simulink model "Swerve_Drive_Example_Model"  (R2023a)
settings: Solver=daessc  StartTime=0.0  StopTime=20  FixedStep=t_sample  RelTol=1e-3
undefined symbols (not defined in the file): t_sample
libraries: Swerve_Modules_Controls_Lib x2, SignalEditorBlockLib x1, Simulation_lib x1
settings Model: SimulationMode=accelerator  Creator=ander  LastModifiedBy=ander

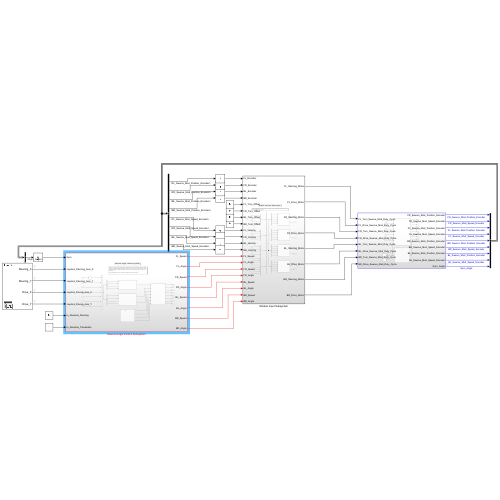
[thumbnail: Simulink's stored preview of the top-level diagram]
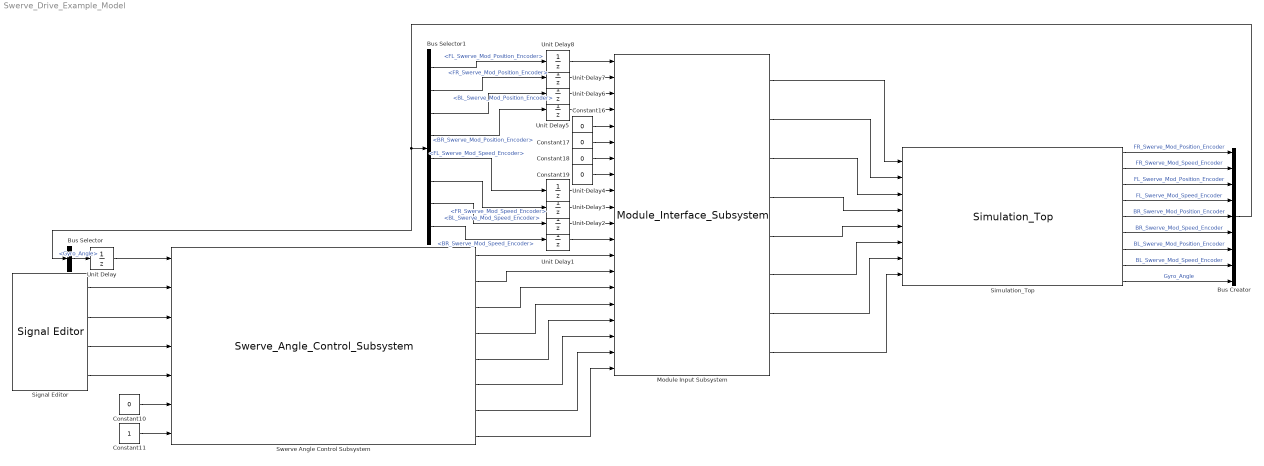
== system Swerve_Drive_Example_Model ==
  Bus Creator : BusCreator  Inputs=9
  Bus Selector : BusSelector  OutputSignals=Gyro_Angle
  Bus Selector1 : BusSelector  OutputSignals=FL_Swerve_Mod_Position_Encoder,FR_Swerve_Mod_Position_Encoder,BL_Swerve_Mod_Position_Encoder,BR_Swerve_Mod_Position_Encoder,FL_Swerve_Mod_Speed_Encoder,FR_Swerve_Mod_Speed_Encoder,BL_Swerve_Mod_Speed_Encoder,BR_Swerve_Mod_Speed_Encoder
  Constant10 : Constant  Value=0  OutDataTypeStr=boolean
  Constant11 : Constant  OutDataTypeStr=boolean
  Constant{16..19} (4 alike) : Constant  Value=0
  Module Input Subsystem : Swerve_Modules_Controls_Lib/Module_Interface_Subsystem  SystemSampleTime=-1  VariantActivationTime=update diagram  Latency=0  AutoFrameSizeCalculation=off
  Signal Editor : SignalEditorBlockLib/Signal Editor  FileName=C:\Users\ander\MATLAB\Projects\SwervePuppy-2.0-VSCODE\simulink\Unit_Tests\Joystick_input_test_data.mat  ActiveScenario=TempTest  ActiveSignal=Drive_X  IsBus=off  OutputBusObjectStr=Bus: BusObject  SampleTime=t_sample  ZeroCross=off  OutputAfterFinalValue=Setting to zero  Unit=inherit  PreserveSignalName=on  ApplySigPropsToAllScenarios=on
  Simulation_Top : Simulation_lib/Simulation_Top  SystemSampleTime=-1  VariantActivationTime=update diagram  Latency=0  AutoFrameSizeCalculation=off
  Swerve Angle Control Subsystem : Swerve_Modules_Controls_Lib/Swerve_Angle_Control_Subsystem  SystemSampleTime=-1  VariantActivationTime=update diagram  Latency=0  AutoFrameSizeCalculation=off
  Unit Delay{,1..8} (9 alike) : UnitDelay  SampleTime=-1  HasFrameUpgradeWarning=on
  wires:
  Constant11/1 -> Swerve Angle Control Subsystem/7
  Constant10/1 -> Swerve Angle Control Subsystem/6
  Constant17/1 -> Module Input Subsystem/6
  Constant19/1 -> Module Input Subsystem/8
  Constant16/1 -> Module Input Subsystem/5
  Constant18/1 -> Module Input Subsystem/7
  Swerve Angle Control Subsystem/4 -> Module Input Subsystem/16
  Swerve Angle Control Subsystem/6 -> Module Input Subsystem/18
  Swerve Angle Control Subsystem/7 -> Module Input Subsystem/19
  Swerve Angle Control Subsystem/2 -> Module Input Subsystem/14
  Swerve Angle Control Subsystem/8 -> Module Input Subsystem/20
  Swerve Angle Control Subsystem/3 -> Module Input Subsystem/15
  Swerve Angle Control Subsystem/1 -> Module Input Subsystem/13
  Swerve Angle Control Subsystem/5 -> Module Input Subsystem/17
  Unit Delay/1 -> Swerve Angle Control Subsystem/1
  Unit Delay1/1 -> Module Input Subsystem/12
  Unit Delay2/1 -> Module Input Subsystem/11
  Unit Delay3/1 -> Module Input Subsystem/10
  Unit Delay4/1 -> Module Input Subsystem/9
  Unit Delay5/1 -> Module Input Subsystem/4
  Unit Delay6/1 -> Module Input Subsystem/3
  Unit Delay7/1 -> Module Input Subsystem/2
  Unit Delay8/1 -> Module Input Subsystem/1
  Simulation_Top/9 -> Bus Creator/9  "Gyro_Angle"
  Simulation_Top/8 -> Bus Creator/8  "BL_Swerve_Mod_Speed_Encoder"
  Simulation_Top/7 -> Bus Creator/7  "BL_Swerve_Mod_Position_Encoder"
  Simulation_Top/6 -> Bus Creator/6  "BR_Swerve_Mod_Speed_Encoder"
  Simulation_Top/5 -> Bus Creator/5  "BR_Swerve_Mod_Position_Encoder"
  Simulation_Top/4 -> Bus Creator/4  "FL_Swerve_Mod_Speed_Encoder"
  Simulation_Top/3 -> Bus Creator/3  "FL_Swerve_Mod_Position_Encoder"
  Simulation_Top/2 -> Bus Creator/2  "FR_Swerve_Mod_Speed_Encoder"
  Simulation_Top/1 -> Bus Creator/1  "FR_Swerve_Mod_Position_Encoder"
  Module Input Subsystem/1 -> Simulation_Top/1
  Module Input Subsystem/2 -> Simulation_Top/2
  Module Input Subsystem/3 -> Simulation_Top/3
  Module Input Subsystem/4 -> Simulation_Top/4
  Module Input Subsystem/5 -> Simulation_Top/5
  Module Input Subsystem/6 -> Simulation_Top/6
  Module Input Subsystem/7 -> Simulation_Top/7
  Module Input Subsystem/8 -> Simulation_Top/8
  Bus Selector/1 -> Unit Delay/1  "<Gyro_Angle>"
  Bus Creator/1 -> Bus Selector/1, Bus Selector1/1
  Bus Selector1/1 -> Unit Delay8/1  "<FL_Swerve_Mod_Position_Encoder>"
  Bus Selector1/2 -> Unit Delay7/1  "<FR_Swerve_Mod_Position_Encoder>"
  Bus Selector1/3 -> Unit Delay6/1  "<BL_Swerve_Mod_Position_Encoder>"
  Bus Selector1/4 -> Unit Delay5/1  "<BR_Swerve_Mod_Position_Encoder>"
  Bus Selector1/5 -> Unit Delay4/1  "<FL_Swerve_Mod_Speed_Encoder>"
  Bus Selector1/6 -> Unit Delay3/1  "<FR_Swerve_Mod_Speed_Encoder>"
  Bus Selector1/7 -> Unit Delay2/1  "<BL_Swerve_Mod_Speed_Encoder>"
  Bus Selector1/8 -> Unit Delay1/1  "<BR_Swerve_Mod_Speed_Encoder>"
  Signal Editor/4 -> Swerve Angle Control Subsystem/5
  Signal Editor/3 -> Swerve Angle Control Subsystem/4
  Signal Editor/2 -> Swerve Angle Control Subsystem/3
  Signal Editor/1 -> Swerve Angle Control Subsystem/2
